simulink model "bld_1125"  (Simulink 2.20)
settings: Solver=ode45  StartTime=0.0  StopTime=10.0  RelTol=1e-3  AbsTol=1e-6
settings Model: ConsistencyChecking=off  RTWPlaceOutputsASAP=off

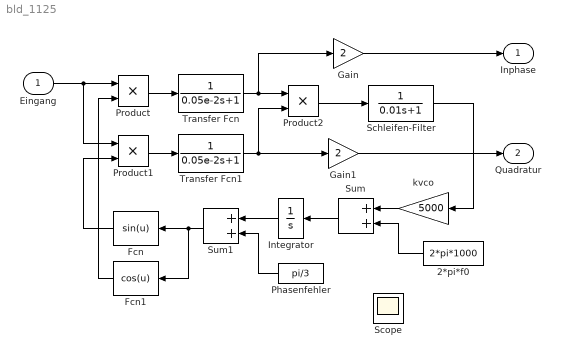
== system bld_1125 ==
  Eingang : Inport  Port=1  PortWidth=-1  SampleTime=-1
  2*pi*f0 : Constant  Orientation=left  Value=2*pi*1000
  Fcn : Fcn  Orientation=left  Expr=sin(u)
  Fcn1 : Fcn  Orientation=left  Expr=cos(u)
  Gain : Gain  Gain=2
  Gain1 : Gain  Gain=2
  Integrator : Integrator  Orientation=left  ExternalReset=none  InitialConditionSource=internal  InitialCondition=0  LimitOutput=off  UpperSaturationLimit=inf  LowerSaturationLimit=-inf  ShowSaturationPort=off  ShowStatePort=off  AbsoluteTolerance=auto
  Phasenfehler : Constant  Orientation=left  Value=pi/3
  Product : Product  Inputs=2
  Product1 : Product  Inputs=2
  Product2 : Product  Inputs=2
  Schleifen-Filter : TransferFcn  Numerator=[1]  Denominator=[0.01 1]
  Scope : Scope
      settings: Floating=on  TickLabels=on  TimeRange=0.1  YMin=-0.125  YMax=0.2  SaveToWorkspace=off  SaveName=ScopeData
  Sum : Sum  Orientation=left  Inputs=++
  Sum1 : Sum  Orientation=left  Inputs=++
  Transfer Fcn : TransferFcn  Numerator=[1]  Denominator="[0.05e-2  1]"
  Transfer Fcn1 : TransferFcn  Numerator=[1]  Denominator="[0.05e-2  1]"
  kvco : Gain  Orientation=left  Gain=5000
  Inphase : Outport  Port=1
  Quadratur : Outport  Port=2
  wires:
  Gain1/1 -> Quadratur/1
  Transfer Fcn1/1 -> Gain1/1, Product2/2
  Gain/1 -> Inphase/1
  Transfer Fcn/1 -> Gain/1, Product2/1
  Fcn1/1 -> Product/2
  Sum1/1 -> Fcn1/1, Fcn/1
  Fcn/1 -> Product1/2
  Schleifen-Filter/1 -> kvco/1
  Product2/1 -> Schleifen-Filter/1
  Product1/1 -> Transfer Fcn1/1
  Product/1 -> Transfer Fcn/1
  Phasenfehler/1 -> Sum1/2
  Integrator/1 -> Sum1/1
  kvco/1 -> Sum/1
  2*pi*f0/1 -> Sum/2
  Sum/1 -> Integrator/1
  Eingang/1 -> Product1/1, Product/1
